simulink model "High_passfilter"  (R2020b)
settings: Solver=VariableStepAuto  StartTime=0.0  StopTime=10.0  RelTol=1e-3
settings Model: Creator=intel  LastModifiedBy=intel

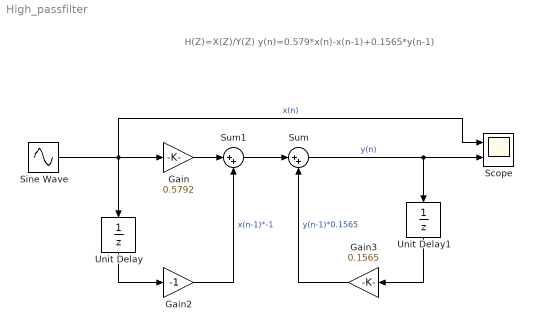
== system High_passfilter ==
  note: H(Z)=X(Z)/Y(Z)
      | y(n)=0.579*x(n)-x(n-1)+0.1565*y(n-1)
  Gain : Gain  Gain=0.5792
  Gain2 : Gain  Gain=-1
  Gain3 : Gain  Gain=0.1565
  Scope : Scope  NumInputPorts=2
  Sine Wave : Sin  Frequency=9999*6.28  SampleTime=0
  Sum : Sum  Inputs=|++
  Sum1 : Sum  Inputs=|++
  Unit Delay : UnitDelay  SampleTime=-1  HasFrameUpgradeWarning=on
  Unit Delay1 : UnitDelay  SampleTime=-1  HasFrameUpgradeWarning=on
  wires:
  Gain/1 -> Sum1/1
  Unit Delay/1 -> Gain2/1
  Unit Delay1/1 -> Gain3/1
  Sum1/1 -> Sum/1
  Gain2/1 -> Sum1/2  "x(n-1)*-1"
  Gain3/1 -> Sum/2  "y(n-1)*0.1565"
  Sum/1 -> Scope/2, Unit Delay1/1  "y(n)"
  Sine Wave/1 -> Scope/1, Unit Delay/1, Gain/1  "x(n)"
